simulink model "PVRobusMPC_final"  (R2018a)
settings: Solver=ode2  StartTime=0.0  StopTime=43200  FixedStep=1  RelTol=1e-3  EnableMultiTasking=on
InitFcn:
  | load PV_model_data
StopFcn:
  | save results Lambda_UV01 T_PV_Reference Tm_f01 Pout01 Tamb Time
  | clear all
  | load results
  | figure
  | subplot(3,1,1)
  | plot(Time./3600,T_PV_Reference,Time./3600,Tm_f01)
  | legend('PV Temperature Reference','PV Temperature')
  | title('MPC Tracking')
  | ylim([350 380])
  | subplot(3,1,2)
  | plot(Time./3600,Lambda_UV01)
  | ylim([250 450])
  | legend('\lambda_U_V')
  | subplot(3,1,3)
  | plot(Time./3600,Pout01)
  | legend('PV Power')
  | xlabel('Time [hours]')
  | ylabel('Watt')
values from neighbouring files (symbols this model uses):
  Global_tilt_Irr_2_2_12_13_5 = [0.000279 0.000786 0.00115 0.00401 0.0047 0.0102 0.011 0.0195 0.0266 0.0299 0.0338 0.0682 ... (2802 elements, 1401x2)]    [PV_model_data.mat]
  Total_light_absorption_in_polystyren = [0.0148235487596 0.0159326919994 0.0170383922491 0.0181406655151 0.0192395277052 0.0203349946285 0.0214270819969 0.0225158054254 0.0236011804327 0.0246832224425 0.0257619467839 0.0264640052027 ... (1151 elements, 1151x1)]    [PV_model_data.mat]
  Total_light_absorption_in_PV_cell_acrylic = [0.0222539070262 0.0239185757929 0.0255780524095 0.0272323791236 0.0288816001883 0.030525761736 0.0321649116541 0.0337990994657 0.0354283762117 0.0370527943369 0.0386724075795 0.0397267002838 ... (1151 elements, 1151x1)]    [PV_model_data.mat]
libraries: mpclib x256
(part 2 of 72)

== system PVRobusMPC_final/4 x 4 x 4 PV Panel 2/4 x 4 PV Panel 6/4 PV Panel 3 ==
  lambda_IR : Inport
  Tambient : Inport  Port=2
  Wind Speed : Inport  Port=3
  Add1 : Sum  Inputs=++++
  Add3 : Sum  Inputs=++++
  PV Panel 5 : Subsystem
  PV Panel 6 : Subsystem
  PV Panel 7 : Subsystem
  PV Panel 8 : Subsystem
  Vout : Outport
  Pout : Outport  Port=2
  wires:
  PV Panel 5/2(Pout) -> Add3/1
  PV Panel 8/2(Pout) -> Add3/4
  Add1/1 -> Vout/1
  PV Panel 8/1(Vout) -> Add1/4
  PV Panel 6/1(Vout) -> Add1/2
  lambda_IR/1 -> PV Panel 5/1(Lambda_IR), PV Panel 7/1(Lambda_IR), PV Panel 8/1(Lambda_IR), PV Panel 6/1(Lambda_IR)
  PV Panel 7/2(Pout) -> Add3/3
  Add3/1 -> Pout/1
  Tambient/1 -> PV Panel 7/2(Tambient), PV Panel 8/2(Tambient), PV Panel 6/2(Tambient), PV Panel 5/2(Tambient)
  Wind Speed/1 -> PV Panel 7/3(Wind Speed), PV Panel 8/3(Wind Speed), PV Panel 6/3(Wind Speed), PV Panel 5/3(Wind Speed)
  PV Panel 7/1(Vout) -> Add1/3
  PV Panel 6/2(Pout) -> Add3/2
  PV Panel 5/1(Vout) -> Add1/1

== system PVRobusMPC_final/4 x 4 x 4 PV Panel 2/4 x 4 PV Panel 6/4 PV Panel 4 ==
  lambda_IR : Inport
  Tambient : Inport  Port=2
  Wind Speed : Inport  Port=3
  Add1 : Sum  Inputs=++++
  Add3 : Sum  Inputs=++++
  PV Panel 5 : Subsystem
  PV Panel 6 : Subsystem
  PV Panel 7 : Subsystem
  PV Panel 8 : Subsystem
  Vout : Outport
  Pout : Outport  Port=2
  wires:
  PV Panel 5/1(Vout) -> Add1/1
  PV Panel 6/2(Pout) -> Add3/2
  PV Panel 7/1(Vout) -> Add1/3
  Wind Speed/1 -> PV Panel 5/3(Wind Speed), PV Panel 6/3(Wind Speed), PV Panel 8/3(Wind Speed), PV Panel 7/3(Wind Speed)
  Tambient/1 -> PV Panel 5/2(Tambient), PV Panel 6/2(Tambient), PV Panel 8/2(Tambient), PV Panel 7/2(Tambient)
  Add3/1 -> Pout/1
  PV Panel 7/2(Pout) -> Add3/3
  lambda_IR/1 -> PV Panel 6/1(Lambda_IR), PV Panel 8/1(Lambda_IR), PV Panel 7/1(Lambda_IR), PV Panel 5/1(Lambda_IR)
  PV Panel 6/1(Vout) -> Add1/2
  PV Panel 8/1(Vout) -> Add1/4
  Add1/1 -> Vout/1
  PV Panel 8/2(Pout) -> Add3/4
  PV Panel 5/2(Pout) -> Add3/1

== system PVRobusMPC_final/4 x 4 x 4 PV Panel 2/4 x 4 PV Panel 7/4 PV Panel 1 ==
  lambda_IR : Inport
  Tambient1 : Inport  Port=2
  Wind Speed : Inport  Port=3
  Add : Sum  Inputs=++++
  Add2 : Sum  Inputs=++++
  PV Panel 1 : Subsystem
  PV Panel 2 : Subsystem
  PV Panel 3 : Subsystem
  PV Panel 4 : Subsystem
  Vout : Outport
  Pout : Outport  Port=2
  wires:
  PV Panel 3/2(Pout) -> Add2/3
  lambda_IR/1 -> PV Panel 1/1(Lambda_IR), PV Panel 2/1(Lambda_IR), PV Panel 4/1(Lambda_IR), PV Panel 3/1(Lambda_IR)
  Add/1 -> Vout/1
  PV Panel 1/2(Pout) -> Add2/1
  Tambient1/1 -> PV Panel 1/2(Tambient), PV Panel 2/2(Tambient), PV Panel 3/2(Tambient), PV Panel 4/2(Tambient)
  PV Panel 1/1(Vout) -> Add/1
  PV Panel 4/1(Vout) -> Add/4
  Wind Speed/1 -> PV Panel 1/3(Wind Speed), PV Panel 2/3(Wind Speed), PV Panel 4/3(Wind Speed), PV Panel 3/3(Wind Speed)
  PV Panel 3/1(Vout) -> Add/3
  PV Panel 2/2(Pout) -> Add2/2
  PV Panel 4/2(Pout) -> Add2/4
  PV Panel 2/1(Vout) -> Add/2
  Add2/1 -> Pout/1

== system PVRobusMPC_final/4 x 4 x 4 PV Panel 2/4 x 4 PV Panel 7/4 PV Panel 2 ==
  lambda_IR : Inport
  Tambient : Inport  Port=2
  Wind Speed : Inport  Port=3
  Add1 : Sum  Inputs=++++
  Add3 : Sum  Inputs=++++
  PV Panel 5 : Subsystem
  PV Panel 6 : Subsystem
  PV Panel 7 : Subsystem
  PV Panel 8 : Subsystem
  Vout : Outport
  Pout : Outport  Port=2
  wires:
  PV Panel 5/1(Vout) -> Add1/1
  PV Panel 6/2(Pout) -> Add3/2
  PV Panel 7/1(Vout) -> Add1/3
  Wind Speed/1 -> PV Panel 5/3(Wind Speed), PV Panel 6/3(Wind Speed), PV Panel 8/3(Wind Speed), PV Panel 7/3(Wind Speed)
  Tambient/1 -> PV Panel 5/2(Tambient), PV Panel 6/2(Tambient), PV Panel 8/2(Tambient), PV Panel 7/2(Tambient)
  Add3/1 -> Pout/1
  PV Panel 7/2(Pout) -> Add3/3
  lambda_IR/1 -> PV Panel 6/1(Lambda_IR), PV Panel 8/1(Lambda_IR), PV Panel 7/1(Lambda_IR), PV Panel 5/1(Lambda_IR)
  PV Panel 6/1(Vout) -> Add1/2
  PV Panel 8/1(Vout) -> Add1/4
  Add1/1 -> Vout/1
  PV Panel 8/2(Pout) -> Add3/4
  PV Panel 5/2(Pout) -> Add3/1

== system PVRobusMPC_final/4 x 4 x 4 PV Panel 2/4 x 4 PV Panel 7/4 PV Panel 3 ==
  lambda_IR : Inport
  Tambient : Inport  Port=2
  Wind Speed : Inport  Port=3
  Add1 : Sum  Inputs=++++
  Add3 : Sum  Inputs=++++
  PV Panel 5 : Subsystem
  PV Panel 6 : Subsystem
  PV Panel 7 : Subsystem
  PV Panel 8 : Subsystem
  Vout : Outport
  Pout : Outport  Port=2
  wires:
  PV Panel 5/2(Pout) -> Add3/1
  PV Panel 8/2(Pout) -> Add3/4
  Add1/1 -> Vout/1
  PV Panel 8/1(Vout) -> Add1/4
  PV Panel 6/1(Vout) -> Add1/2
  lambda_IR/1 -> PV Panel 5/1(Lambda_IR), PV Panel 7/1(Lambda_IR), PV Panel 8/1(Lambda_IR), PV Panel 6/1(Lambda_IR)
  PV Panel 7/2(Pout) -> Add3/3
  Add3/1 -> Pout/1
  Tambient/1 -> PV Panel 7/2(Tambient), PV Panel 8/2(Tambient), PV Panel 6/2(Tambient), PV Panel 5/2(Tambient)
  Wind Speed/1 -> PV Panel 7/3(Wind Speed), PV Panel 8/3(Wind Speed), PV Panel 6/3(Wind Speed), PV Panel 5/3(Wind Speed)
  PV Panel 7/1(Vout) -> Add1/3
  PV Panel 6/2(Pout) -> Add3/2
  PV Panel 5/1(Vout) -> Add1/1

== system PVRobusMPC_final/4 x 4 x 4 PV Panel 2/4 x 4 PV Panel 7/4 PV Panel 4 ==
  lambda_IR : Inport
  Tambient : Inport  Port=2
  Wind Speed : Inport  Port=3
  Add1 : Sum  Inputs=++++
  Add3 : Sum  Inputs=++++
  PV Panel 5 : Subsystem
  PV Panel 6 : Subsystem
  PV Panel 7 : Subsystem
  PV Panel 8 : Subsystem
  Vout : Outport
  Pout : Outport  Port=2
  wires:
  PV Panel 5/1(Vout) -> Add1/1
  PV Panel 6/2(Pout) -> Add3/2
  PV Panel 7/1(Vout) -> Add1/3
  Wind Speed/1 -> PV Panel 5/3(Wind Speed), PV Panel 6/3(Wind Speed), PV Panel 8/3(Wind Speed), PV Panel 7/3(Wind Speed)
  Tambient/1 -> PV Panel 5/2(Tambient), PV Panel 6/2(Tambient), PV Panel 8/2(Tambient), PV Panel 7/2(Tambient)
  Add3/1 -> Pout/1
  PV Panel 7/2(Pout) -> Add3/3
  lambda_IR/1 -> PV Panel 6/1(Lambda_IR), PV Panel 8/1(Lambda_IR), PV Panel 7/1(Lambda_IR), PV Panel 5/1(Lambda_IR)
  PV Panel 6/1(Vout) -> Add1/2
  PV Panel 8/1(Vout) -> Add1/4
  Add1/1 -> Vout/1
  PV Panel 8/2(Pout) -> Add3/4
  PV Panel 5/2(Pout) -> Add3/1

== system PVRobusMPC_final/4 x 4 x 4 PV Panel 2/4 x 4 PV Panel 8/4 PV Panel 1 ==
  lambda_IR : Inport
  Tambient1 : Inport  Port=2
  Wind Speed : Inport  Port=3
  Add : Sum  Inputs=++++
  Add2 : Sum  Inputs=++++
  PV Panel 1 : Subsystem
  PV Panel 2 : Subsystem
  PV Panel 3 : Subsystem
  PV Panel 4 : Subsystem
  Vout : Outport
  Pout : Outport  Port=2
  wires:
  Add2/1 -> Pout/1
  PV Panel 2/1(Vout) -> Add/2
  PV Panel 4/2(Pout) -> Add2/4
  PV Panel 2/2(Pout) -> Add2/2
  PV Panel 3/1(Vout) -> Add/3
  Wind Speed/1 -> PV Panel 3/3(Wind Speed), PV Panel 4/3(Wind Speed), PV Panel 2/3(Wind Speed), PV Panel 1/3(Wind Speed)
  PV Panel 4/1(Vout) -> Add/4
  PV Panel 1/1(Vout) -> Add/1
  Tambient1/1 -> PV Panel 4/2(Tambient), PV Panel 3/2(Tambient), PV Panel 2/2(Tambient), PV Panel 1/2(Tambient)
  PV Panel 1/2(Pout) -> Add2/1
  Add/1 -> Vout/1
  lambda_IR/1 -> PV Panel 3/1(Lambda_IR), PV Panel 4/1(Lambda_IR), PV Panel 2/1(Lambda_IR), PV Panel 1/1(Lambda_IR)
  PV Panel 3/2(Pout) -> Add2/3

== system PVRobusMPC_final/4 x 4 x 4 PV Panel 2/4 x 4 PV Panel 8/4 PV Panel 2 ==
  lambda_IR : Inport
  Tambient : Inport  Port=2
  Wind Speed : Inport  Port=3
  Add1 : Sum  Inputs=++++
  Add3 : Sum  Inputs=++++
  PV Panel 5 : Subsystem
  PV Panel 6 : Subsystem
  PV Panel 7 : Subsystem
  PV Panel 8 : Subsystem
  Vout : Outport
  Pout : Outport  Port=2
  wires:
  PV Panel 5/2(Pout) -> Add3/1
  PV Panel 8/2(Pout) -> Add3/4
  Add1/1 -> Vout/1
  PV Panel 8/1(Vout) -> Add1/4
  PV Panel 6/1(Vout) -> Add1/2
  lambda_IR/1 -> PV Panel 5/1(Lambda_IR), PV Panel 7/1(Lambda_IR), PV Panel 8/1(Lambda_IR), PV Panel 6/1(Lambda_IR)
  PV Panel 7/2(Pout) -> Add3/3
  Add3/1 -> Pout/1
  Tambient/1 -> PV Panel 7/2(Tambient), PV Panel 8/2(Tambient), PV Panel 6/2(Tambient), PV Panel 5/2(Tambient)
  Wind Speed/1 -> PV Panel 7/3(Wind Speed), PV Panel 8/3(Wind Speed), PV Panel 6/3(Wind Speed), PV Panel 5/3(Wind Speed)
  PV Panel 7/1(Vout) -> Add1/3
  PV Panel 6/2(Pout) -> Add3/2
  PV Panel 5/1(Vout) -> Add1/1

== system PVRobusMPC_final/4 x 4 x 4 PV Panel 2/4 x 4 PV Panel 8/4 PV Panel 3 ==
  lambda_IR : Inport
  Tambient : Inport  Port=2
  Wind Speed : Inport  Port=3
  Add1 : Sum  Inputs=++++
  Add3 : Sum  Inputs=++++
  PV Panel 5 : Subsystem
  PV Panel 6 : Subsystem
  PV Panel 7 : Subsystem
  PV Panel 8 : Subsystem
  Vout : Outport
  Pout : Outport  Port=2
  wires:
  PV Panel 5/1(Vout) -> Add1/1
  PV Panel 6/2(Pout) -> Add3/2
  PV Panel 7/1(Vout) -> Add1/3
  Wind Speed/1 -> PV Panel 5/3(Wind Speed), PV Panel 6/3(Wind Speed), PV Panel 8/3(Wind Speed), PV Panel 7/3(Wind Speed)
  Tambient/1 -> PV Panel 5/2(Tambient), PV Panel 6/2(Tambient), PV Panel 8/2(Tambient), PV Panel 7/2(Tambient)
  Add3/1 -> Pout/1
  PV Panel 7/2(Pout) -> Add3/3
  lambda_IR/1 -> PV Panel 6/1(Lambda_IR), PV Panel 8/1(Lambda_IR), PV Panel 7/1(Lambda_IR), PV Panel 5/1(Lambda_IR)
  PV Panel 6/1(Vout) -> Add1/2
  PV Panel 8/1(Vout) -> Add1/4
  Add1/1 -> Vout/1
  PV Panel 8/2(Pout) -> Add3/4
  PV Panel 5/2(Pout) -> Add3/1

== system PVRobusMPC_final/4 x 4 x 4 PV Panel 2/4 x 4 PV Panel 8/4 PV Panel 4 ==
  lambda_IR : Inport
  Tambient : Inport  Port=2
  Wind Speed : Inport  Port=3
  Add1 : Sum  Inputs=++++
  Add3 : Sum  Inputs=++++
  PV Panel 5 : Subsystem
  PV Panel 6 : Subsystem
  PV Panel 7 : Subsystem
  PV Panel 8 : Subsystem
  Vout : Outport
  Pout : Outport  Port=2
  wires:
  PV Panel 5/2(Pout) -> Add3/1
  PV Panel 8/2(Pout) -> Add3/4
  Add1/1 -> Vout/1
  PV Panel 8/1(Vout) -> Add1/4
  PV Panel 6/1(Vout) -> Add1/2
  lambda_IR/1 -> PV Panel 5/1(Lambda_IR), PV Panel 7/1(Lambda_IR), PV Panel 8/1(Lambda_IR), PV Panel 6/1(Lambda_IR)
  PV Panel 7/2(Pout) -> Add3/3
  Add3/1 -> Pout/1
  Tambient/1 -> PV Panel 7/2(Tambient), PV Panel 8/2(Tambient), PV Panel 6/2(Tambient), PV Panel 5/2(Tambient)
  Wind Speed/1 -> PV Panel 7/3(Wind Speed), PV Panel 8/3(Wind Speed), PV Panel 6/3(Wind Speed), PV Panel 5/3(Wind Speed)
  PV Panel 7/1(Vout) -> Add1/3
  PV Panel 6/2(Pout) -> Add3/2
  PV Panel 5/1(Vout) -> Add1/1

== system PVRobusMPC_final/4 x 4 x 4 PV Panel 3/4 x 4 PV Panel 5/4 PV Panel 1 ==
  lambda_IR : Inport
  Tambient1 : Inport  Port=2
  Wind Speed : Inport  Port=3
  Add : Sum  Inputs=++++
  Add2 : Sum  Inputs=++++
  PV Panel 1 : Subsystem
  PV Panel 2 : Subsystem
  PV Panel 3 : Subsystem
  PV Panel 4 : Subsystem
  Vout : Outport
  Pout : Outport  Port=2
  wires:
  Add2/1 -> Pout/1
  PV Panel 2/1(Vout) -> Add/2
  PV Panel 4/2(Pout) -> Add2/4
  PV Panel 2/2(Pout) -> Add2/2
  PV Panel 3/1(Vout) -> Add/3
  Wind Speed/1 -> PV Panel 3/3(Wind Speed), PV Panel 4/3(Wind Speed), PV Panel 2/3(Wind Speed), PV Panel 1/3(Wind Speed)
  PV Panel 4/1(Vout) -> Add/4
  PV Panel 1/1(Vout) -> Add/1
  Tambient1/1 -> PV Panel 4/2(Tambient), PV Panel 3/2(Tambient), PV Panel 2/2(Tambient), PV Panel 1/2(Tambient)
  PV Panel 1/2(Pout) -> Add2/1
  Add/1 -> Vout/1
  lambda_IR/1 -> PV Panel 3/1(Lambda_IR), PV Panel 4/1(Lambda_IR), PV Panel 2/1(Lambda_IR), PV Panel 1/1(Lambda_IR)
  PV Panel 3/2(Pout) -> Add2/3

== system PVRobusMPC_final/4 x 4 x 4 PV Panel 3/4 x 4 PV Panel 5/4 PV Panel 2 ==
  lambda_IR : Inport
  Tambient : Inport  Port=2
  Wind Speed : Inport  Port=3
  Add1 : Sum  Inputs=++++
  Add3 : Sum  Inputs=++++
  PV Panel 5 : Subsystem
  PV Panel 6 : Subsystem
  PV Panel 7 : Subsystem
  PV Panel 8 : Subsystem
  Vout : Outport
  Pout : Outport  Port=2
  wires:
  PV Panel 5/2(Pout) -> Add3/1
  PV Panel 8/2(Pout) -> Add3/4
  Add1/1 -> Vout/1
  PV Panel 8/1(Vout) -> Add1/4
  PV Panel 6/1(Vout) -> Add1/2
  lambda_IR/1 -> PV Panel 5/1(Lambda_IR), PV Panel 7/1(Lambda_IR), PV Panel 8/1(Lambda_IR), PV Panel 6/1(Lambda_IR)
  PV Panel 7/2(Pout) -> Add3/3
  Add3/1 -> Pout/1
  Tambient/1 -> PV Panel 7/2(Tambient), PV Panel 8/2(Tambient), PV Panel 6/2(Tambient), PV Panel 5/2(Tambient)
  Wind Speed/1 -> PV Panel 7/3(Wind Speed), PV Panel 8/3(Wind Speed), PV Panel 6/3(Wind Speed), PV Panel 5/3(Wind Speed)
  PV Panel 7/1(Vout) -> Add1/3
  PV Panel 6/2(Pout) -> Add3/2
  PV Panel 5/1(Vout) -> Add1/1

== system PVRobusMPC_final/4 x 4 x 4 PV Panel 3/4 x 4 PV Panel 5/4 PV Panel 3 ==
  lambda_IR : Inport
  Tambient : Inport  Port=2
  Wind Speed : Inport  Port=3
  Add1 : Sum  Inputs=++++
  Add3 : Sum  Inputs=++++
  PV Panel 5 : Subsystem
  PV Panel 6 : Subsystem
  PV Panel 7 : Subsystem
  PV Panel 8 : Subsystem
  Vout : Outport
  Pout : Outport  Port=2
  wires:
  PV Panel 5/1(Vout) -> Add1/1
  PV Panel 6/2(Pout) -> Add3/2
  PV Panel 7/1(Vout) -> Add1/3
  Wind Speed/1 -> PV Panel 5/3(Wind Speed), PV Panel 6/3(Wind Speed), PV Panel 8/3(Wind Speed), PV Panel 7/3(Wind Speed)
  Tambient/1 -> PV Panel 5/2(Tambient), PV Panel 6/2(Tambient), PV Panel 8/2(Tambient), PV Panel 7/2(Tambient)
  Add3/1 -> Pout/1
  PV Panel 7/2(Pout) -> Add3/3
  lambda_IR/1 -> PV Panel 6/1(Lambda_IR), PV Panel 8/1(Lambda_IR), PV Panel 7/1(Lambda_IR), PV Panel 5/1(Lambda_IR)
  PV Panel 6/1(Vout) -> Add1/2
  PV Panel 8/1(Vout) -> Add1/4
  Add1/1 -> Vout/1
  PV Panel 8/2(Pout) -> Add3/4
  PV Panel 5/2(Pout) -> Add3/1

== system PVRobusMPC_final/4 x 4 x 4 PV Panel 3/4 x 4 PV Panel 5/4 PV Panel 4 ==
  lambda_IR : Inport
  Tambient : Inport  Port=2
  Wind Speed : Inport  Port=3
  Add1 : Sum  Inputs=++++
  Add3 : Sum  Inputs=++++
  PV Panel 5 : Subsystem
  PV Panel 6 : Subsystem
  PV Panel 7 : Subsystem
  PV Panel 8 : Subsystem
  Vout : Outport
  Pout : Outport  Port=2
  wires:
  PV Panel 5/2(Pout) -> Add3/1
  PV Panel 8/2(Pout) -> Add3/4
  Add1/1 -> Vout/1
  PV Panel 8/1(Vout) -> Add1/4
  PV Panel 6/1(Vout) -> Add1/2
  lambda_IR/1 -> PV Panel 5/1(Lambda_IR), PV Panel 7/1(Lambda_IR), PV Panel 8/1(Lambda_IR), PV Panel 6/1(Lambda_IR)
  PV Panel 7/2(Pout) -> Add3/3
  Add3/1 -> Pout/1
  Tambient/1 -> PV Panel 7/2(Tambient), PV Panel 8/2(Tambient), PV Panel 6/2(Tambient), PV Panel 5/2(Tambient)
  Wind Speed/1 -> PV Panel 7/3(Wind Speed), PV Panel 8/3(Wind Speed), PV Panel 6/3(Wind Speed), PV Panel 5/3(Wind Speed)
  PV Panel 7/1(Vout) -> Add1/3
  PV Panel 6/2(Pout) -> Add3/2
  PV Panel 5/1(Vout) -> Add1/1

== system PVRobusMPC_final/4 x 4 x 4 PV Panel 3/4 x 4 PV Panel 6/4 PV Panel 1 ==
  lambda_IR : Inport
  Tambient1 : Inport  Port=2
  Wind Speed : Inport  Port=3
  Add : Sum  Inputs=++++
  Add2 : Sum  Inputs=++++
  PV Panel 1 : Subsystem
  PV Panel 2 : Subsystem
  PV Panel 3 : Subsystem
  PV Panel 4 : Subsystem
  Vout : Outport
  Pout : Outport  Port=2
  wires:
  Add2/1 -> Pout/1
  PV Panel 2/1(Vout) -> Add/2
  PV Panel 4/2(Pout) -> Add2/4
  PV Panel 2/2(Pout) -> Add2/2
  PV Panel 3/1(Vout) -> Add/3
  Wind Speed/1 -> PV Panel 3/3(Wind Speed), PV Panel 4/3(Wind Speed), PV Panel 2/3(Wind Speed), PV Panel 1/3(Wind Speed)
  PV Panel 4/1(Vout) -> Add/4
  PV Panel 1/1(Vout) -> Add/1
  Tambient1/1 -> PV Panel 4/2(Tambient), PV Panel 3/2(Tambient), PV Panel 2/2(Tambient), PV Panel 1/2(Tambient)
  PV Panel 1/2(Pout) -> Add2/1
  Add/1 -> Vout/1
  lambda_IR/1 -> PV Panel 3/1(Lambda_IR), PV Panel 4/1(Lambda_IR), PV Panel 2/1(Lambda_IR), PV Panel 1/1(Lambda_IR)
  PV Panel 3/2(Pout) -> Add2/3

== system PVRobusMPC_final/4 x 4 x 4 PV Panel 3/4 x 4 PV Panel 6/4 PV Panel 2 ==
  lambda_IR : Inport
  Tambient : Inport  Port=2
  Wind Speed : Inport  Port=3
  Add1 : Sum  Inputs=++++
  Add3 : Sum  Inputs=++++
  PV Panel 5 : Subsystem
  PV Panel 6 : Subsystem
  PV Panel 7 : Subsystem
  PV Panel 8 : Subsystem
  Vout : Outport
  Pout : Outport  Port=2
  wires:
  PV Panel 5/2(Pout) -> Add3/1
  PV Panel 8/2(Pout) -> Add3/4
  Add1/1 -> Vout/1
  PV Panel 8/1(Vout) -> Add1/4
  PV Panel 6/1(Vout) -> Add1/2
  lambda_IR/1 -> PV Panel 5/1(Lambda_IR), PV Panel 7/1(Lambda_IR), PV Panel 8/1(Lambda_IR), PV Panel 6/1(Lambda_IR)
  PV Panel 7/2(Pout) -> Add3/3
  Add3/1 -> Pout/1
  Tambient/1 -> PV Panel 7/2(Tambient), PV Panel 8/2(Tambient), PV Panel 6/2(Tambient), PV Panel 5/2(Tambient)
  Wind Speed/1 -> PV Panel 7/3(Wind Speed), PV Panel 8/3(Wind Speed), PV Panel 6/3(Wind Speed), PV Panel 5/3(Wind Speed)
  PV Panel 7/1(Vout) -> Add1/3
  PV Panel 6/2(Pout) -> Add3/2
  PV Panel 5/1(Vout) -> Add1/1

== system PVRobusMPC_final/4 x 4 x 4 PV Panel 3/4 x 4 PV Panel 6/4 PV Panel 3 ==
  lambda_IR : Inport
  Tambient : Inport  Port=2
  Wind Speed : Inport  Port=3
  Add1 : Sum  Inputs=++++
  Add3 : Sum  Inputs=++++
  PV Panel 5 : Subsystem
  PV Panel 6 : Subsystem
  PV Panel 7 : Subsystem
  PV Panel 8 : Subsystem
  Vout : Outport
  Pout : Outport  Port=2
  wires:
  PV Panel 5/1(Vout) -> Add1/1
  PV Panel 6/2(Pout) -> Add3/2
  PV Panel 7/1(Vout) -> Add1/3
  Wind Speed/1 -> PV Panel 5/3(Wind Speed), PV Panel 6/3(Wind Speed), PV Panel 8/3(Wind Speed), PV Panel 7/3(Wind Speed)
  Tambient/1 -> PV Panel 5/2(Tambient), PV Panel 6/2(Tambient), PV Panel 8/2(Tambient), PV Panel 7/2(Tambient)
  Add3/1 -> Pout/1
  PV Panel 7/2(Pout) -> Add3/3
  lambda_IR/1 -> PV Panel 6/1(Lambda_IR), PV Panel 8/1(Lambda_IR), PV Panel 7/1(Lambda_IR), PV Panel 5/1(Lambda_IR)
  PV Panel 6/1(Vout) -> Add1/2
  PV Panel 8/1(Vout) -> Add1/4
  Add1/1 -> Vout/1
  PV Panel 8/2(Pout) -> Add3/4
  PV Panel 5/2(Pout) -> Add3/1

== system PVRobusMPC_final/4 x 4 x 4 PV Panel 3/4 x 4 PV Panel 6/4 PV Panel 4 ==
  lambda_IR : Inport
  Tambient : Inport  Port=2
  Wind Speed : Inport  Port=3
  Add1 : Sum  Inputs=++++
  Add3 : Sum  Inputs=++++
  PV Panel 5 : Subsystem
  PV Panel 6 : Subsystem
  PV Panel 7 : Subsystem
  PV Panel 8 : Subsystem
  Vout : Outport
  Pout : Outport  Port=2
  wires:
  PV Panel 5/2(Pout) -> Add3/1
  PV Panel 8/2(Pout) -> Add3/4
  Add1/1 -> Vout/1
  PV Panel 8/1(Vout) -> Add1/4
  PV Panel 6/1(Vout) -> Add1/2
  lambda_IR/1 -> PV Panel 5/1(Lambda_IR), PV Panel 7/1(Lambda_IR), PV Panel 8/1(Lambda_IR), PV Panel 6/1(Lambda_IR)
  PV Panel 7/2(Pout) -> Add3/3
  Add3/1 -> Pout/1
  Tambient/1 -> PV Panel 7/2(Tambient), PV Panel 8/2(Tambient), PV Panel 6/2(Tambient), PV Panel 5/2(Tambient)
  Wind Speed/1 -> PV Panel 7/3(Wind Speed), PV Panel 8/3(Wind Speed), PV Panel 6/3(Wind Speed), PV Panel 5/3(Wind Speed)
  PV Panel 7/1(Vout) -> Add1/3
  PV Panel 6/2(Pout) -> Add3/2
  PV Panel 5/1(Vout) -> Add1/1

== system PVRobusMPC_final/4 x 4 x 4 PV Panel 3/4 x 4 PV Panel 7/4 PV Panel 1 ==
  lambda_IR : Inport
  Tambient1 : Inport  Port=2
  Wind Speed : Inport  Port=3
  Add : Sum  Inputs=++++
  Add2 : Sum  Inputs=++++
  PV Panel 1 : Subsystem
  PV Panel 2 : Subsystem
  PV Panel 3 : Subsystem
  PV Panel 4 : Subsystem
  Vout : Outport
  Pout : Outport  Port=2
  wires:
  Add2/1 -> Pout/1
  PV Panel 2/1(Vout) -> Add/2
  PV Panel 4/2(Pout) -> Add2/4
  PV Panel 2/2(Pout) -> Add2/2
  PV Panel 3/1(Vout) -> Add/3
  Wind Speed/1 -> PV Panel 3/3(Wind Speed), PV Panel 4/3(Wind Speed), PV Panel 2/3(Wind Speed), PV Panel 1/3(Wind Speed)
  PV Panel 4/1(Vout) -> Add/4
  PV Panel 1/1(Vout) -> Add/1
  Tambient1/1 -> PV Panel 4/2(Tambient), PV Panel 3/2(Tambient), PV Panel 2/2(Tambient), PV Panel 1/2(Tambient)
  PV Panel 1/2(Pout) -> Add2/1
  Add/1 -> Vout/1
  lambda_IR/1 -> PV Panel 3/1(Lambda_IR), PV Panel 4/1(Lambda_IR), PV Panel 2/1(Lambda_IR), PV Panel 1/1(Lambda_IR)
  PV Panel 3/2(Pout) -> Add2/3

== system PVRobusMPC_final/4 x 4 x 4 PV Panel 3/4 x 4 PV Panel 7/4 PV Panel 2 ==
  lambda_IR : Inport
  Tambient : Inport  Port=2
  Wind Speed : Inport  Port=3
  Add1 : Sum  Inputs=++++
  Add3 : Sum  Inputs=++++
  PV Panel 5 : Subsystem
  PV Panel 6 : Subsystem
  PV Panel 7 : Subsystem
  PV Panel 8 : Subsystem
  Vout : Outport
  Pout : Outport  Port=2
  wires:
  PV Panel 5/2(Pout) -> Add3/1
  PV Panel 8/2(Pout) -> Add3/4
  Add1/1 -> Vout/1
  PV Panel 8/1(Vout) -> Add1/4
  PV Panel 6/1(Vout) -> Add1/2
  lambda_IR/1 -> PV Panel 5/1(Lambda_IR), PV Panel 7/1(Lambda_IR), PV Panel 8/1(Lambda_IR), PV Panel 6/1(Lambda_IR)
  PV Panel 7/2(Pout) -> Add3/3
  Add3/1 -> Pout/1
  Tambient/1 -> PV Panel 7/2(Tambient), PV Panel 8/2(Tambient), PV Panel 6/2(Tambient), PV Panel 5/2(Tambient)
  Wind Speed/1 -> PV Panel 7/3(Wind Speed), PV Panel 8/3(Wind Speed), PV Panel 6/3(Wind Speed), PV Panel 5/3(Wind Speed)
  PV Panel 7/1(Vout) -> Add1/3
  PV Panel 6/2(Pout) -> Add3/2
  PV Panel 5/1(Vout) -> Add1/1

== system PVRobusMPC_final/4 x 4 x 4 PV Panel 3/4 x 4 PV Panel 7/4 PV Panel 3 ==
  lambda_IR : Inport
  Tambient : Inport  Port=2
  Wind Speed : Inport  Port=3
  Add1 : Sum  Inputs=++++
  Add3 : Sum  Inputs=++++
  PV Panel 5 : Subsystem
  PV Panel 6 : Subsystem
  PV Panel 7 : Subsystem
  PV Panel 8 : Subsystem
  Vout : Outport
  Pout : Outport  Port=2
  wires:
  PV Panel 5/1(Vout) -> Add1/1
  PV Panel 6/2(Pout) -> Add3/2
  PV Panel 7/1(Vout) -> Add1/3
  Wind Speed/1 -> PV Panel 5/3(Wind Speed), PV Panel 6/3(Wind Speed), PV Panel 8/3(Wind Speed), PV Panel 7/3(Wind Speed)
  Tambient/1 -> PV Panel 5/2(Tambient), PV Panel 6/2(Tambient), PV Panel 8/2(Tambient), PV Panel 7/2(Tambient)
  Add3/1 -> Pout/1
  PV Panel 7/2(Pout) -> Add3/3
  lambda_IR/1 -> PV Panel 6/1(Lambda_IR), PV Panel 8/1(Lambda_IR), PV Panel 7/1(Lambda_IR), PV Panel 5/1(Lambda_IR)
  PV Panel 6/1(Vout) -> Add1/2
  PV Panel 8/1(Vout) -> Add1/4
  Add1/1 -> Vout/1
  PV Panel 8/2(Pout) -> Add3/4
  PV Panel 5/2(Pout) -> Add3/1

== system PVRobusMPC_final/4 x 4 x 4 PV Panel 3/4 x 4 PV Panel 7/4 PV Panel 4 ==
  lambda_IR : Inport
  Tambient : Inport  Port=2
  Wind Speed : Inport  Port=3
  Add1 : Sum  Inputs=++++
  Add3 : Sum  Inputs=++++
  PV Panel 5 : Subsystem
  PV Panel 6 : Subsystem
  PV Panel 7 : Subsystem
  PV Panel 8 : Subsystem
  Vout : Outport
  Pout : Outport  Port=2
  wires:
  PV Panel 5/2(Pout) -> Add3/1
  PV Panel 8/2(Pout) -> Add3/4
  Add1/1 -> Vout/1
  PV Panel 8/1(Vout) -> Add1/4
  PV Panel 6/1(Vout) -> Add1/2
  lambda_IR/1 -> PV Panel 5/1(Lambda_IR), PV Panel 7/1(Lambda_IR), PV Panel 8/1(Lambda_IR), PV Panel 6/1(Lambda_IR)
  PV Panel 7/2(Pout) -> Add3/3
  Add3/1 -> Pout/1
  Tambient/1 -> PV Panel 7/2(Tambient), PV Panel 8/2(Tambient), PV Panel 6/2(Tambient), PV Panel 5/2(Tambient)
  Wind Speed/1 -> PV Panel 7/3(Wind Speed), PV Panel 8/3(Wind Speed), PV Panel 6/3(Wind Speed), PV Panel 5/3(Wind Speed)
  PV Panel 7/1(Vout) -> Add1/3
  PV Panel 6/2(Pout) -> Add3/2
  PV Panel 5/1(Vout) -> Add1/1

== system PVRobusMPC_final/4 x 4 x 4 PV Panel 3/4 x 4 PV Panel 8/4 PV Panel 1 ==
  lambda_IR : Inport
  Tambient1 : Inport  Port=2
  Wind Speed : Inport  Port=3
  Add : Sum  Inputs=++++
  Add2 : Sum  Inputs=++++
  PV Panel 1 : Subsystem
  PV Panel 2 : Subsystem
  PV Panel 3 : Subsystem
  PV Panel 4 : Subsystem
  Vout : Outport
  Pout : Outport  Port=2
  wires:
  PV Panel 3/2(Pout) -> Add2/3
  lambda_IR/1 -> PV Panel 1/1(Lambda_IR), PV Panel 2/1(Lambda_IR), PV Panel 4/1(Lambda_IR), PV Panel 3/1(Lambda_IR)
  Add/1 -> Vout/1
  PV Panel 1/2(Pout) -> Add2/1
  Tambient1/1 -> PV Panel 1/2(Tambient), PV Panel 2/2(Tambient), PV Panel 3/2(Tambient), PV Panel 4/2(Tambient)
  PV Panel 1/1(Vout) -> Add/1
  PV Panel 4/1(Vout) -> Add/4
  Wind Speed/1 -> PV Panel 1/3(Wind Speed), PV Panel 2/3(Wind Speed), PV Panel 4/3(Wind Speed), PV Panel 3/3(Wind Speed)
  PV Panel 3/1(Vout) -> Add/3
  PV Panel 2/2(Pout) -> Add2/2
  PV Panel 4/2(Pout) -> Add2/4
  PV Panel 2/1(Vout) -> Add/2
  Add2/1 -> Pout/1

== system PVRobusMPC_final/4 x 4 x 4 PV Panel 3/4 x 4 PV Panel 8/4 PV Panel 2 ==
  lambda_IR : Inport
  Tambient : Inport  Port=2
  Wind Speed : Inport  Port=3
  Add1 : Sum  Inputs=++++
  Add3 : Sum  Inputs=++++
  PV Panel 5 : Subsystem
  PV Panel 6 : Subsystem
  PV Panel 7 : Subsystem
  PV Panel 8 : Subsystem
  Vout : Outport
  Pout : Outport  Port=2
  wires:
  PV Panel 5/1(Vout) -> Add1/1
  PV Panel 6/2(Pout) -> Add3/2
  PV Panel 7/1(Vout) -> Add1/3
  Wind Speed/1 -> PV Panel 5/3(Wind Speed), PV Panel 6/3(Wind Speed), PV Panel 8/3(Wind Speed), PV Panel 7/3(Wind Speed)
  Tambient/1 -> PV Panel 5/2(Tambient), PV Panel 6/2(Tambient), PV Panel 8/2(Tambient), PV Panel 7/2(Tambient)
  Add3/1 -> Pout/1
  PV Panel 7/2(Pout) -> Add3/3
  lambda_IR/1 -> PV Panel 6/1(Lambda_IR), PV Panel 8/1(Lambda_IR), PV Panel 7/1(Lambda_IR), PV Panel 5/1(Lambda_IR)
  PV Panel 6/1(Vout) -> Add1/2
  PV Panel 8/1(Vout) -> Add1/4
  Add1/1 -> Vout/1
  PV Panel 8/2(Pout) -> Add3/4
  PV Panel 5/2(Pout) -> Add3/1

== system PVRobusMPC_final/4 x 4 x 4 PV Panel 3/4 x 4 PV Panel 8/4 PV Panel 3 ==
  lambda_IR : Inport
  Tambient : Inport  Port=2
  Wind Speed : Inport  Port=3
  Add1 : Sum  Inputs=++++
  Add3 : Sum  Inputs=++++
  PV Panel 5 : Subsystem
  PV Panel 6 : Subsystem
  PV Panel 7 : Subsystem
  PV Panel 8 : Subsystem
  Vout : Outport
  Pout : Outport  Port=2
  wires:
  PV Panel 5/2(Pout) -> Add3/1
  PV Panel 8/2(Pout) -> Add3/4
  Add1/1 -> Vout/1
  PV Panel 8/1(Vout) -> Add1/4
  PV Panel 6/1(Vout) -> Add1/2
  lambda_IR/1 -> PV Panel 5/1(Lambda_IR), PV Panel 7/1(Lambda_IR), PV Panel 8/1(Lambda_IR), PV Panel 6/1(Lambda_IR)
  PV Panel 7/2(Pout) -> Add3/3
  Add3/1 -> Pout/1
  Tambient/1 -> PV Panel 7/2(Tambient), PV Panel 8/2(Tambient), PV Panel 6/2(Tambient), PV Panel 5/2(Tambient)
  Wind Speed/1 -> PV Panel 7/3(Wind Speed), PV Panel 8/3(Wind Speed), PV Panel 6/3(Wind Speed), PV Panel 5/3(Wind Speed)
  PV Panel 7/1(Vout) -> Add1/3
  PV Panel 6/2(Pout) -> Add3/2
  PV Panel 5/1(Vout) -> Add1/1

== system PVRobusMPC_final/4 x 4 x 4 PV Panel 3/4 x 4 PV Panel 8/4 PV Panel 4 ==
  lambda_IR : Inport
  Tambient : Inport  Port=2
  Wind Speed : Inport  Port=3
  Add1 : Sum  Inputs=++++
  Add3 : Sum  Inputs=++++
  PV Panel 5 : Subsystem
  PV Panel 6 : Subsystem
  PV Panel 7 : Subsystem
  PV Panel 8 : Subsystem
  Vout : Outport
  Pout : Outport  Port=2
  wires:
  PV Panel 5/1(Vout) -> Add1/1
  PV Panel 6/2(Pout) -> Add3/2
  PV Panel 7/1(Vout) -> Add1/3
  Wind Speed/1 -> PV Panel 5/3(Wind Speed), PV Panel 6/3(Wind Speed), PV Panel 8/3(Wind Speed), PV Panel 7/3(Wind Speed)
  Tambient/1 -> PV Panel 5/2(Tambient), PV Panel 6/2(Tambient), PV Panel 8/2(Tambient), PV Panel 7/2(Tambient)
  Add3/1 -> Pout/1
  PV Panel 7/2(Pout) -> Add3/3
  lambda_IR/1 -> PV Panel 6/1(Lambda_IR), PV Panel 8/1(Lambda_IR), PV Panel 7/1(Lambda_IR), PV Panel 5/1(Lambda_IR)
  PV Panel 6/1(Vout) -> Add1/2
  PV Panel 8/1(Vout) -> Add1/4
  Add1/1 -> Vout/1
  PV Panel 8/2(Pout) -> Add3/4
  PV Panel 5/2(Pout) -> Add3/1

== system PVRobusMPC_final/4 x 4 x 4 PV Panel 4/4 x 4 PV Panel 5/4 PV Panel 1 ==
  lambda_IR : Inport
  Tambient1 : Inport  Port=2
  Wind Speed : Inport  Port=3
  Add : Sum  Inputs=++++
  Add2 : Sum  Inputs=++++
  PV Panel 1 : Subsystem
  PV Panel 2 : Subsystem
  PV Panel 3 : Subsystem
  PV Panel 4 : Subsystem
  Vout : Outport
  Pout : Outport  Port=2
  wires:
  PV Panel 3/2(Pout) -> Add2/3
  lambda_IR/1 -> PV Panel 1/1(Lambda_IR), PV Panel 2/1(Lambda_IR), PV Panel 4/1(Lambda_IR), PV Panel 3/1(Lambda_IR)
  Add/1 -> Vout/1
  PV Panel 1/2(Pout) -> Add2/1
  Tambient1/1 -> PV Panel 1/2(Tambient), PV Panel 2/2(Tambient), PV Panel 3/2(Tambient), PV Panel 4/2(Tambient)
  PV Panel 1/1(Vout) -> Add/1
  PV Panel 4/1(Vout) -> Add/4
  Wind Speed/1 -> PV Panel 1/3(Wind Speed), PV Panel 2/3(Wind Speed), PV Panel 4/3(Wind Speed), PV Panel 3/3(Wind Speed)
  PV Panel 3/1(Vout) -> Add/3
  PV Panel 2/2(Pout) -> Add2/2
  PV Panel 4/2(Pout) -> Add2/4
  PV Panel 2/1(Vout) -> Add/2
  Add2/1 -> Pout/1

== system PVRobusMPC_final/4 x 4 x 4 PV Panel 4/4 x 4 PV Panel 5/4 PV Panel 2 ==
  lambda_IR : Inport
  Tambient : Inport  Port=2
  Wind Speed : Inport  Port=3
  Add1 : Sum  Inputs=++++
  Add3 : Sum  Inputs=++++
  PV Panel 5 : Subsystem
  PV Panel 6 : Subsystem
  PV Panel 7 : Subsystem
  PV Panel 8 : Subsystem
  Vout : Outport
  Pout : Outport  Port=2
  wires:
  PV Panel 5/1(Vout) -> Add1/1
  PV Panel 6/2(Pout) -> Add3/2
  PV Panel 7/1(Vout) -> Add1/3
  Wind Speed/1 -> PV Panel 5/3(Wind Speed), PV Panel 6/3(Wind Speed), PV Panel 8/3(Wind Speed), PV Panel 7/3(Wind Speed)
  Tambient/1 -> PV Panel 5/2(Tambient), PV Panel 6/2(Tambient), PV Panel 8/2(Tambient), PV Panel 7/2(Tambient)
  Add3/1 -> Pout/1
  PV Panel 7/2(Pout) -> Add3/3
  lambda_IR/1 -> PV Panel 6/1(Lambda_IR), PV Panel 8/1(Lambda_IR), PV Panel 7/1(Lambda_IR), PV Panel 5/1(Lambda_IR)
  PV Panel 6/1(Vout) -> Add1/2
  PV Panel 8/1(Vout) -> Add1/4
  Add1/1 -> Vout/1
  PV Panel 8/2(Pout) -> Add3/4
  PV Panel 5/2(Pout) -> Add3/1

== system PVRobusMPC_final/4 x 4 x 4 PV Panel 4/4 x 4 PV Panel 5/4 PV Panel 3 ==
  lambda_IR : Inport
  Tambient : Inport  Port=2
  Wind Speed : Inport  Port=3
  Add1 : Sum  Inputs=++++
  Add3 : Sum  Inputs=++++
  PV Panel 5 : Subsystem
  PV Panel 6 : Subsystem
  PV Panel 7 : Subsystem
  PV Panel 8 : Subsystem
  Vout : Outport
  Pout : Outport  Port=2
  wires:
  PV Panel 5/2(Pout) -> Add3/1
  PV Panel 8/2(Pout) -> Add3/4
  Add1/1 -> Vout/1
  PV Panel 8/1(Vout) -> Add1/4
  PV Panel 6/1(Vout) -> Add1/2
  lambda_IR/1 -> PV Panel 5/1(Lambda_IR), PV Panel 7/1(Lambda_IR), PV Panel 8/1(Lambda_IR), PV Panel 6/1(Lambda_IR)
  PV Panel 7/2(Pout) -> Add3/3
  Add3/1 -> Pout/1
  Tambient/1 -> PV Panel 7/2(Tambient), PV Panel 8/2(Tambient), PV Panel 6/2(Tambient), PV Panel 5/2(Tambient)
  Wind Speed/1 -> PV Panel 7/3(Wind Speed), PV Panel 8/3(Wind Speed), PV Panel 6/3(Wind Speed), PV Panel 5/3(Wind Speed)
  PV Panel 7/1(Vout) -> Add1/3
  PV Panel 6/2(Pout) -> Add3/2
  PV Panel 5/1(Vout) -> Add1/1

== system PVRobusMPC_final/4 x 4 x 4 PV Panel 4/4 x 4 PV Panel 5/4 PV Panel 4 ==
  lambda_IR : Inport
  Tambient : Inport  Port=2
  Wind Speed : Inport  Port=3
  Add1 : Sum  Inputs=++++
  Add3 : Sum  Inputs=++++
  PV Panel 5 : Subsystem
  PV Panel 6 : Subsystem
  PV Panel 7 : Subsystem
  PV Panel 8 : Subsystem
  Vout : Outport
  Pout : Outport  Port=2
  wires:
  PV Panel 5/1(Vout) -> Add1/1
  PV Panel 6/2(Pout) -> Add3/2
  PV Panel 7/1(Vout) -> Add1/3
  Wind Speed/1 -> PV Panel 5/3(Wind Speed), PV Panel 6/3(Wind Speed), PV Panel 8/3(Wind Speed), PV Panel 7/3(Wind Speed)
  Tambient/1 -> PV Panel 5/2(Tambient), PV Panel 6/2(Tambient), PV Panel 8/2(Tambient), PV Panel 7/2(Tambient)
  Add3/1 -> Pout/1
  PV Panel 7/2(Pout) -> Add3/3
  lambda_IR/1 -> PV Panel 6/1(Lambda_IR), PV Panel 8/1(Lambda_IR), PV Panel 7/1(Lambda_IR), PV Panel 5/1(Lambda_IR)
  PV Panel 6/1(Vout) -> Add1/2
  PV Panel 8/1(Vout) -> Add1/4
  Add1/1 -> Vout/1
  PV Panel 8/2(Pout) -> Add3/4
  PV Panel 5/2(Pout) -> Add3/1

== system PVRobusMPC_final/4 x 4 x 4 PV Panel 4/4 x 4 PV Panel 6/4 PV Panel 1 ==
  lambda_IR : Inport
  Tambient1 : Inport  Port=2
  Wind Speed : Inport  Port=3
  Add : Sum  Inputs=++++
  Add2 : Sum  Inputs=++++
  PV Panel 1 : Subsystem
  PV Panel 2 : Subsystem
  PV Panel 3 : Subsystem
  PV Panel 4 : Subsystem
  Vout : Outport
  Pout : Outport  Port=2
  wires:
  PV Panel 3/2(Pout) -> Add2/3
  lambda_IR/1 -> PV Panel 1/1(Lambda_IR), PV Panel 2/1(Lambda_IR), PV Panel 4/1(Lambda_IR), PV Panel 3/1(Lambda_IR)
  Add/1 -> Vout/1
  PV Panel 1/2(Pout) -> Add2/1
  Tambient1/1 -> PV Panel 1/2(Tambient), PV Panel 2/2(Tambient), PV Panel 3/2(Tambient), PV Panel 4/2(Tambient)
  PV Panel 1/1(Vout) -> Add/1
  PV Panel 4/1(Vout) -> Add/4
  Wind Speed/1 -> PV Panel 1/3(Wind Speed), PV Panel 2/3(Wind Speed), PV Panel 4/3(Wind Speed), PV Panel 3/3(Wind Speed)
  PV Panel 3/1(Vout) -> Add/3
  PV Panel 2/2(Pout) -> Add2/2
  PV Panel 4/2(Pout) -> Add2/4
  PV Panel 2/1(Vout) -> Add/2
  Add2/1 -> Pout/1

== system PVRobusMPC_final/4 x 4 x 4 PV Panel 4/4 x 4 PV Panel 6/4 PV Panel 2 ==
  lambda_IR : Inport
  Tambient : Inport  Port=2
  Wind Speed : Inport  Port=3
  Add1 : Sum  Inputs=++++
  Add3 : Sum  Inputs=++++
  PV Panel 5 : Subsystem
  PV Panel 6 : Subsystem
  PV Panel 7 : Subsystem
  PV Panel 8 : Subsystem
  Vout : Outport
  Pout : Outport  Port=2
  wires:
  PV Panel 5/1(Vout) -> Add1/1
  PV Panel 6/2(Pout) -> Add3/2
  PV Panel 7/1(Vout) -> Add1/3
  Wind Speed/1 -> PV Panel 5/3(Wind Speed), PV Panel 6/3(Wind Speed), PV Panel 8/3(Wind Speed), PV Panel 7/3(Wind Speed)
  Tambient/1 -> PV Panel 5/2(Tambient), PV Panel 6/2(Tambient), PV Panel 8/2(Tambient), PV Panel 7/2(Tambient)
  Add3/1 -> Pout/1
  PV Panel 7/2(Pout) -> Add3/3
  lambda_IR/1 -> PV Panel 6/1(Lambda_IR), PV Panel 8/1(Lambda_IR), PV Panel 7/1(Lambda_IR), PV Panel 5/1(Lambda_IR)
  PV Panel 6/1(Vout) -> Add1/2
  PV Panel 8/1(Vout) -> Add1/4
  Add1/1 -> Vout/1
  PV Panel 8/2(Pout) -> Add3/4
  PV Panel 5/2(Pout) -> Add3/1

== system PVRobusMPC_final/4 x 4 x 4 PV Panel 4/4 x 4 PV Panel 6/4 PV Panel 3 ==
  lambda_IR : Inport
  Tambient : Inport  Port=2
  Wind Speed : Inport  Port=3
  Add1 : Sum  Inputs=++++
  Add3 : Sum  Inputs=++++
  PV Panel 5 : Subsystem
  PV Panel 6 : Subsystem
  PV Panel 7 : Subsystem
  PV Panel 8 : Subsystem
  Vout : Outport
  Pout : Outport  Port=2
  wires:
  PV Panel 5/2(Pout) -> Add3/1
  PV Panel 8/2(Pout) -> Add3/4
  Add1/1 -> Vout/1
  PV Panel 8/1(Vout) -> Add1/4
  PV Panel 6/1(Vout) -> Add1/2
  lambda_IR/1 -> PV Panel 5/1(Lambda_IR), PV Panel 7/1(Lambda_IR), PV Panel 8/1(Lambda_IR), PV Panel 6/1(Lambda_IR)
  PV Panel 7/2(Pout) -> Add3/3
  Add3/1 -> Pout/1
  Tambient/1 -> PV Panel 7/2(Tambient), PV Panel 8/2(Tambient), PV Panel 6/2(Tambient), PV Panel 5/2(Tambient)
  Wind Speed/1 -> PV Panel 7/3(Wind Speed), PV Panel 8/3(Wind Speed), PV Panel 6/3(Wind Speed), PV Panel 5/3(Wind Speed)
  PV Panel 7/1(Vout) -> Add1/3
  PV Panel 6/2(Pout) -> Add3/2
  PV Panel 5/1(Vout) -> Add1/1

== system PVRobusMPC_final/4 x 4 x 4 PV Panel 4/4 x 4 PV Panel 6/4 PV Panel 4 ==
  lambda_IR : Inport
  Tambient : Inport  Port=2
  Wind Speed : Inport  Port=3
  Add1 : Sum  Inputs=++++
  Add3 : Sum  Inputs=++++
  PV Panel 5 : Subsystem
  PV Panel 6 : Subsystem
  PV Panel 7 : Subsystem
  PV Panel 8 : Subsystem
  Vout : Outport
  Pout : Outport  Port=2
  wires:
  PV Panel 5/1(Vout) -> Add1/1
  PV Panel 6/2(Pout) -> Add3/2
  PV Panel 7/1(Vout) -> Add1/3
  Wind Speed/1 -> PV Panel 5/3(Wind Speed), PV Panel 6/3(Wind Speed), PV Panel 8/3(Wind Speed), PV Panel 7/3(Wind Speed)
  Tambient/1 -> PV Panel 5/2(Tambient), PV Panel 6/2(Tambient), PV Panel 8/2(Tambient), PV Panel 7/2(Tambient)
  Add3/1 -> Pout/1
  PV Panel 7/2(Pout) -> Add3/3
  lambda_IR/1 -> PV Panel 6/1(Lambda_IR), PV Panel 8/1(Lambda_IR), PV Panel 7/1(Lambda_IR), PV Panel 5/1(Lambda_IR)
  PV Panel 6/1(Vout) -> Add1/2
  PV Panel 8/1(Vout) -> Add1/4
  Add1/1 -> Vout/1
  PV Panel 8/2(Pout) -> Add3/4
  PV Panel 5/2(Pout) -> Add3/1

== system PVRobusMPC_final/4 x 4 x 4 PV Panel 4/4 x 4 PV Panel 7/4 PV Panel 1 ==
  lambda_IR : Inport
  Tambient1 : Inport  Port=2
  Wind Speed : Inport  Port=3
  Add : Sum  Inputs=++++
  Add2 : Sum  Inputs=++++
  PV Panel 1 : Subsystem
  PV Panel 2 : Subsystem
  PV Panel 3 : Subsystem
  PV Panel 4 : Subsystem
  Vout : Outport
  Pout : Outport  Port=2
  wires:
  PV Panel 3/2(Pout) -> Add2/3
  lambda_IR/1 -> PV Panel 1/1(Lambda_IR), PV Panel 2/1(Lambda_IR), PV Panel 4/1(Lambda_IR), PV Panel 3/1(Lambda_IR)
  Add/1 -> Vout/1
  PV Panel 1/2(Pout) -> Add2/1
  Tambient1/1 -> PV Panel 1/2(Tambient), PV Panel 2/2(Tambient), PV Panel 3/2(Tambient), PV Panel 4/2(Tambient)
  PV Panel 1/1(Vout) -> Add/1
  PV Panel 4/1(Vout) -> Add/4
  Wind Speed/1 -> PV Panel 1/3(Wind Speed), PV Panel 2/3(Wind Speed), PV Panel 4/3(Wind Speed), PV Panel 3/3(Wind Speed)
  PV Panel 3/1(Vout) -> Add/3
  PV Panel 2/2(Pout) -> Add2/2
  PV Panel 4/2(Pout) -> Add2/4
  PV Panel 2/1(Vout) -> Add/2
  Add2/1 -> Pout/1

== system PVRobusMPC_final/4 x 4 x 4 PV Panel 4/4 x 4 PV Panel 7/4 PV Panel 2 ==
  lambda_IR : Inport
  Tambient : Inport  Port=2
  Wind Speed : Inport  Port=3
  Add1 : Sum  Inputs=++++
  Add3 : Sum  Inputs=++++
  PV Panel 5 : Subsystem
  PV Panel 6 : Subsystem
  PV Panel 7 : Subsystem
  PV Panel 8 : Subsystem
  Vout : Outport
  Pout : Outport  Port=2
  wires:
  PV Panel 5/1(Vout) -> Add1/1
  PV Panel 6/2(Pout) -> Add3/2
  PV Panel 7/1(Vout) -> Add1/3
  Wind Speed/1 -> PV Panel 5/3(Wind Speed), PV Panel 6/3(Wind Speed), PV Panel 8/3(Wind Speed), PV Panel 7/3(Wind Speed)
  Tambient/1 -> PV Panel 5/2(Tambient), PV Panel 6/2(Tambient), PV Panel 8/2(Tambient), PV Panel 7/2(Tambient)
  Add3/1 -> Pout/1
  PV Panel 7/2(Pout) -> Add3/3
  lambda_IR/1 -> PV Panel 6/1(Lambda_IR), PV Panel 8/1(Lambda_IR), PV Panel 7/1(Lambda_IR), PV Panel 5/1(Lambda_IR)
  PV Panel 6/1(Vout) -> Add1/2
  PV Panel 8/1(Vout) -> Add1/4
  Add1/1 -> Vout/1
  PV Panel 8/2(Pout) -> Add3/4
  PV Panel 5/2(Pout) -> Add3/1

== system PVRobusMPC_final/4 x 4 x 4 PV Panel 4/4 x 4 PV Panel 7/4 PV Panel 3 ==
  lambda_IR : Inport
  Tambient : Inport  Port=2
  Wind Speed : Inport  Port=3
  Add1 : Sum  Inputs=++++
  Add3 : Sum  Inputs=++++
  PV Panel 5 : Subsystem
  PV Panel 6 : Subsystem
  PV Panel 7 : Subsystem
  PV Panel 8 : Subsystem
  Vout : Outport
  Pout : Outport  Port=2
  wires:
  PV Panel 5/2(Pout) -> Add3/1
  PV Panel 8/2(Pout) -> Add3/4
  Add1/1 -> Vout/1
  PV Panel 8/1(Vout) -> Add1/4
  PV Panel 6/1(Vout) -> Add1/2
  lambda_IR/1 -> PV Panel 5/1(Lambda_IR), PV Panel 7/1(Lambda_IR), PV Panel 8/1(Lambda_IR), PV Panel 6/1(Lambda_IR)
  PV Panel 7/2(Pout) -> Add3/3
  Add3/1 -> Pout/1
  Tambient/1 -> PV Panel 7/2(Tambient), PV Panel 8/2(Tambient), PV Panel 6/2(Tambient), PV Panel 5/2(Tambient)
  Wind Speed/1 -> PV Panel 7/3(Wind Speed), PV Panel 8/3(Wind Speed), PV Panel 6/3(Wind Speed), PV Panel 5/3(Wind Speed)
  PV Panel 7/1(Vout) -> Add1/3
  PV Panel 6/2(Pout) -> Add3/2
  PV Panel 5/1(Vout) -> Add1/1

== system PVRobusMPC_final/4 x 4 x 4 PV Panel 4/4 x 4 PV Panel 7/4 PV Panel 4 ==
  lambda_IR : Inport
  Tambient : Inport  Port=2
  Wind Speed : Inport  Port=3
  Add1 : Sum  Inputs=++++
  Add3 : Sum  Inputs=++++
  PV Panel 5 : Subsystem
  PV Panel 6 : Subsystem
  PV Panel 7 : Subsystem
  PV Panel 8 : Subsystem
  Vout : Outport
  Pout : Outport  Port=2
  wires:
  PV Panel 5/1(Vout) -> Add1/1
  PV Panel 6/2(Pout) -> Add3/2
  PV Panel 7/1(Vout) -> Add1/3
  Wind Speed/1 -> PV Panel 5/3(Wind Speed), PV Panel 6/3(Wind Speed), PV Panel 8/3(Wind Speed), PV Panel 7/3(Wind Speed)
  Tambient/1 -> PV Panel 5/2(Tambient), PV Panel 6/2(Tambient), PV Panel 8/2(Tambient), PV Panel 7/2(Tambient)
  Add3/1 -> Pout/1
  PV Panel 7/2(Pout) -> Add3/3
  lambda_IR/1 -> PV Panel 6/1(Lambda_IR), PV Panel 8/1(Lambda_IR), PV Panel 7/1(Lambda_IR), PV Panel 5/1(Lambda_IR)
  PV Panel 6/1(Vout) -> Add1/2
  PV Panel 8/1(Vout) -> Add1/4
  Add1/1 -> Vout/1
  PV Panel 8/2(Pout) -> Add3/4
  PV Panel 5/2(Pout) -> Add3/1

== system PVRobusMPC_final/4 x 4 x 4 PV Panel 4/4 x 4 PV Panel 8/4 PV Panel 1 ==
  lambda_IR : Inport
  Tambient1 : Inport  Port=2
  Wind Speed : Inport  Port=3
  Add : Sum  Inputs=++++
  Add2 : Sum  Inputs=++++
  PV Panel 1 : Subsystem
  PV Panel 2 : Subsystem
  PV Panel 3 : Subsystem
  PV Panel 4 : Subsystem
  Vout : Outport
  Pout : Outport  Port=2
  wires:
  Add2/1 -> Pout/1
  PV Panel 2/1(Vout) -> Add/2
  PV Panel 4/2(Pout) -> Add2/4
  PV Panel 2/2(Pout) -> Add2/2
  PV Panel 3/1(Vout) -> Add/3
  Wind Speed/1 -> PV Panel 3/3(Wind Speed), PV Panel 4/3(Wind Speed), PV Panel 2/3(Wind Speed), PV Panel 1/3(Wind Speed)
  PV Panel 4/1(Vout) -> Add/4
  PV Panel 1/1(Vout) -> Add/1
  Tambient1/1 -> PV Panel 4/2(Tambient), PV Panel 3/2(Tambient), PV Panel 2/2(Tambient), PV Panel 1/2(Tambient)
  PV Panel 1/2(Pout) -> Add2/1
  Add/1 -> Vout/1
  lambda_IR/1 -> PV Panel 3/1(Lambda_IR), PV Panel 4/1(Lambda_IR), PV Panel 2/1(Lambda_IR), PV Panel 1/1(Lambda_IR)
  PV Panel 3/2(Pout) -> Add2/3

== system PVRobusMPC_final/4 x 4 x 4 PV Panel 4/4 x 4 PV Panel 8/4 PV Panel 2 ==
  lambda_IR : Inport
  Tambient : Inport  Port=2
  Wind Speed : Inport  Port=3
  Add1 : Sum  Inputs=++++
  Add3 : Sum  Inputs=++++
  PV Panel 5 : Subsystem
  PV Panel 6 : Subsystem
  PV Panel 7 : Subsystem
  PV Panel 8 : Subsystem
  Vout : Outport
  Pout : Outport  Port=2
  wires:
  PV Panel 5/2(Pout) -> Add3/1
  PV Panel 8/2(Pout) -> Add3/4
  Add1/1 -> Vout/1
  PV Panel 8/1(Vout) -> Add1/4
  PV Panel 6/1(Vout) -> Add1/2
  lambda_IR/1 -> PV Panel 5/1(Lambda_IR), PV Panel 7/1(Lambda_IR), PV Panel 8/1(Lambda_IR), PV Panel 6/1(Lambda_IR)
  PV Panel 7/2(Pout) -> Add3/3
  Add3/1 -> Pout/1
  Tambient/1 -> PV Panel 7/2(Tambient), PV Panel 8/2(Tambient), PV Panel 6/2(Tambient), PV Panel 5/2(Tambient)
  Wind Speed/1 -> PV Panel 7/3(Wind Speed), PV Panel 8/3(Wind Speed), PV Panel 6/3(Wind Speed), PV Panel 5/3(Wind Speed)
  PV Panel 7/1(Vout) -> Add1/3
  PV Panel 6/2(Pout) -> Add3/2
  PV Panel 5/1(Vout) -> Add1/1

== system PVRobusMPC_final/4 x 4 x 4 PV Panel 4/4 x 4 PV Panel 8/4 PV Panel 3 ==
  lambda_IR : Inport
  Tambient : Inport  Port=2
  Wind Speed : Inport  Port=3
  Add1 : Sum  Inputs=++++
  Add3 : Sum  Inputs=++++
  PV Panel 5 : Subsystem
  PV Panel 6 : Subsystem
  PV Panel 7 : Subsystem
  PV Panel 8 : Subsystem
  Vout : Outport
  Pout : Outport  Port=2
  wires:
  PV Panel 5/1(Vout) -> Add1/1
  PV Panel 6/2(Pout) -> Add3/2
  PV Panel 7/1(Vout) -> Add1/3
  Wind Speed/1 -> PV Panel 5/3(Wind Speed), PV Panel 6/3(Wind Speed), PV Panel 8/3(Wind Speed), PV Panel 7/3(Wind Speed)
  Tambient/1 -> PV Panel 5/2(Tambient), PV Panel 6/2(Tambient), PV Panel 8/2(Tambient), PV Panel 7/2(Tambient)
  Add3/1 -> Pout/1
  PV Panel 7/2(Pout) -> Add3/3
  lambda_IR/1 -> PV Panel 6/1(Lambda_IR), PV Panel 8/1(Lambda_IR), PV Panel 7/1(Lambda_IR), PV Panel 5/1(Lambda_IR)
  PV Panel 6/1(Vout) -> Add1/2
  PV Panel 8/1(Vout) -> Add1/4
  Add1/1 -> Vout/1
  PV Panel 8/2(Pout) -> Add3/4
  PV Panel 5/2(Pout) -> Add3/1

== system PVRobusMPC_final/4 x 4 x 4 PV Panel 4/4 x 4 PV Panel 8/4 PV Panel 4 ==
  lambda_IR : Inport
  Tambient : Inport  Port=2
  Wind Speed : Inport  Port=3
  Add1 : Sum  Inputs=++++
  Add3 : Sum  Inputs=++++
  PV Panel 5 : Subsystem
  PV Panel 6 : Subsystem
  PV Panel 7 : Subsystem
  PV Panel 8 : Subsystem
  Vout : Outport
  Pout : Outport  Port=2
  wires:
  PV Panel 5/2(Pout) -> Add3/1
  PV Panel 8/2(Pout) -> Add3/4
  Add1/1 -> Vout/1
  PV Panel 8/1(Vout) -> Add1/4
  PV Panel 6/1(Vout) -> Add1/2
  lambda_IR/1 -> PV Panel 5/1(Lambda_IR), PV Panel 7/1(Lambda_IR), PV Panel 8/1(Lambda_IR), PV Panel 6/1(Lambda_IR)
  PV Panel 7/2(Pout) -> Add3/3
  Add3/1 -> Pout/1
  Tambient/1 -> PV Panel 7/2(Tambient), PV Panel 8/2(Tambient), PV Panel 6/2(Tambient), PV Panel 5/2(Tambient)
  Wind Speed/1 -> PV Panel 7/3(Wind Speed), PV Panel 8/3(Wind Speed), PV Panel 6/3(Wind Speed), PV Panel 5/3(Wind Speed)
  PV Panel 7/1(Vout) -> Add1/3
  PV Panel 6/2(Pout) -> Add3/2
  PV Panel 5/1(Vout) -> Add1/1

== system PVRobusMPC_final/4 x 4 x 4 PV Panel 1/4 x 4 PV Panel 1/4 PV Panel 1/PV Panel 1 ==
  Lambda_IR : Inport
  Tambient : Inport  Port=2
  Wind Speed : Inport  Port=3
  PV MPC : Subsystem
  Photovolatic Panel : Subsystem  mask{Temp_Initial=380}
      mask prompts: Temp_Initial "Initial Temperature in C"
  To Workspace : ToWorkspace  VariableName=Tm_f01  SampleTime=1
  To Workspace1 : ToWorkspace  VariableName=Pout01  SampleTime=1
  To Workspace2 : ToWorkspace  VariableName=Lambda_UV01  SampleTime=1
  Unit Delay : UnitDelay  InitialCondition=380
  Unit Delay1 : UnitDelay  InitialCondition=4
  Vout : Outport
  Pout : Outport  Port=2
  wires:
  Unit Delay/1 -> PV MPC/1(Tm_f), To Workspace/1
  PV MPC/1(Lambda_UV) -> To Workspace2/1, Photovolatic Panel/1(Lambda_UV)
  Unit Delay1/1 -> Pout/1, To Workspace1/1
  Lambda_IR/1 -> Photovolatic Panel/2(Lambda_IR)
  Photovolatic Panel/3(Vout [Volts]) -> Vout/1
  Tambient/1 -> PV MPC/2(Tambient), Photovolatic Panel/3(Tambient)
  Photovolatic Panel/2(Pout [Watt]) -> Unit Delay1/1
  Photovolatic Panel/1(Tm_f [K]) -> Unit Delay/1
  Wind Speed/1 -> Photovolatic Panel/4(WS)

== system PVRobusMPC_final/4 x 4 x 4 PV Panel 1/4 x 4 PV Panel 1/4 PV Panel 1/PV Panel 2 ==
  Lambda_IR : Inport
  Tambient : Inport  Port=2
  Wind Speed : Inport  Port=3
  PV MPC : Subsystem
  Photovolatic Panel : Subsystem  mask{Temp_Initial=380}
      mask prompts: Temp_Initial "Initial Temperature in C"
  Unit Delay : UnitDelay  InitialCondition=380
  Unit Delay1 : UnitDelay  InitialCondition=4
  Vout : Outport
  Pout : Outport  Port=2
  wires:
  Wind Speed/1 -> Photovolatic Panel/4(WS)
  Photovolatic Panel/1(Tm_f [K]) -> Unit Delay/1
  Photovolatic Panel/2(Pout [Watt]) -> Unit Delay1/1
  Tambient/1 -> Photovolatic Panel/3(Tambient), PV MPC/2(Tambient)
  Photovolatic Panel/3(Vout [Volts]) -> Vout/1
  Lambda_IR/1 -> Photovolatic Panel/2(Lambda_IR)
  Unit Delay1/1 -> Pout/1
  PV MPC/1(Lambda_UV) -> Photovolatic Panel/1(Lambda_UV)
  Unit Delay/1 -> PV MPC/1(Tm_f)

== system PVRobusMPC_final/4 x 4 x 4 PV Panel 1/4 x 4 PV Panel 1/4 PV Panel 1/PV Panel 3 ==
  Lambda_IR : Inport
  Tambient : Inport  Port=2
  Wind Speed : Inport  Port=3
  PV MPC : Subsystem
  Photovolatic Panel : Subsystem  mask{Temp_Initial=380}
      mask prompts: Temp_Initial "Initial Temperature in C"
  Unit Delay : UnitDelay  InitialCondition=380
  Unit Delay1 : UnitDelay  InitialCondition=4
  Vout : Outport
  Pout : Outport  Port=2
  wires:
  Unit Delay/1 -> PV MPC/1(Tm_f)
  PV MPC/1(Lambda_UV) -> Photovolatic Panel/1(Lambda_UV)
  Unit Delay1/1 -> Pout/1
  Lambda_IR/1 -> Photovolatic Panel/2(Lambda_IR)
  Photovolatic Panel/3(Vout [Volts]) -> Vout/1
  Tambient/1 -> PV MPC/2(Tambient), Photovolatic Panel/3(Tambient)
  Photovolatic Panel/2(Pout [Watt]) -> Unit Delay1/1
  Photovolatic Panel/1(Tm_f [K]) -> Unit Delay/1
  Wind Speed/1 -> Photovolatic Panel/4(WS)

== system PVRobusMPC_final/4 x 4 x 4 PV Panel 1/4 x 4 PV Panel 1/4 PV Panel 1/PV Panel 4 ==
  Lambda_IR : Inport
  Tambient : Inport  Port=2
  Wind Speed : Inport  Port=3
  PV MPC : Subsystem
  Photovolatic Panel : Subsystem  mask{Temp_Initial=380}
      mask prompts: Temp_Initial "Initial Temperature in C"
  Unit Delay : UnitDelay  InitialCondition=380
  Unit Delay1 : UnitDelay  InitialCondition=4
  Vout : Outport
  Pout : Outport  Port=2
  wires:
  Wind Speed/1 -> Photovolatic Panel/4(WS)
  Photovolatic Panel/1(Tm_f [K]) -> Unit Delay/1
  Photovolatic Panel/2(Pout [Watt]) -> Unit Delay1/1
  Tambient/1 -> Photovolatic Panel/3(Tambient), PV MPC/2(Tambient)
  Photovolatic Panel/3(Vout [Volts]) -> Vout/1
  Lambda_IR/1 -> Photovolatic Panel/2(Lambda_IR)
  Unit Delay1/1 -> Pout/1
  PV MPC/1(Lambda_UV) -> Photovolatic Panel/1(Lambda_UV)
  Unit Delay/1 -> PV MPC/1(Tm_f)

== system PVRobusMPC_final/4 x 4 x 4 PV Panel 1/4 x 4 PV Panel 1/4 PV Panel 2/PV Panel 5 ==
  Lambda_IR : Inport
  Tambient : Inport  Port=2
  Wind Speed : Inport  Port=3
  PV MPC : Subsystem
  Photovolatic Panel : Subsystem  mask{Temp_Initial=380}
      mask prompts: Temp_Initial "Initial Temperature in C"
  Unit Delay : UnitDelay  InitialCondition=380
  Unit Delay1 : UnitDelay  InitialCondition=4
  Vout : Outport
  Pout : Outport  Port=2
  wires:
  Unit Delay/1 -> PV MPC/1(Tm_f)
  PV MPC/1(Lambda_UV) -> Photovolatic Panel/1(Lambda_UV)
  Unit Delay1/1 -> Pout/1
  Lambda_IR/1 -> Photovolatic Panel/2(Lambda_IR)
  Photovolatic Panel/3(Vout [Volts]) -> Vout/1
  Tambient/1 -> PV MPC/2(Tambient), Photovolatic Panel/3(Tambient)
  Photovolatic Panel/2(Pout [Watt]) -> Unit Delay1/1
  Photovolatic Panel/1(Tm_f [K]) -> Unit Delay/1
  Wind Speed/1 -> Photovolatic Panel/4(WS)

== system PVRobusMPC_final/4 x 4 x 4 PV Panel 1/4 x 4 PV Panel 1/4 PV Panel 2/PV Panel 6 ==
  Lambda_IR : Inport
  Tambient : Inport  Port=2
  Wind Speed : Inport  Port=3
  PV MPC : Subsystem
  Photovolatic Panel : Subsystem  mask{Temp_Initial=380}
      mask prompts: Temp_Initial "Initial Temperature in C"
  Unit Delay : UnitDelay  InitialCondition=380
  Unit Delay1 : UnitDelay  InitialCondition=4
  Vout : Outport
  Pout : Outport  Port=2
  wires:
  Wind Speed/1 -> Photovolatic Panel/4(WS)
  Photovolatic Panel/1(Tm_f [K]) -> Unit Delay/1
  Photovolatic Panel/2(Pout [Watt]) -> Unit Delay1/1
  Tambient/1 -> Photovolatic Panel/3(Tambient), PV MPC/2(Tambient)
  Photovolatic Panel/3(Vout [Volts]) -> Vout/1
  Lambda_IR/1 -> Photovolatic Panel/2(Lambda_IR)
  Unit Delay1/1 -> Pout/1
  PV MPC/1(Lambda_UV) -> Photovolatic Panel/1(Lambda_UV)
  Unit Delay/1 -> PV MPC/1(Tm_f)

== system PVRobusMPC_final/4 x 4 x 4 PV Panel 1/4 x 4 PV Panel 1/4 PV Panel 2/PV Panel 7 ==
  Lambda_IR : Inport
  Tambient : Inport  Port=2
  Wind Speed : Inport  Port=3
  PV MPC : Subsystem
  Photovolatic Panel : Subsystem  mask{Temp_Initial=380}
      mask prompts: Temp_Initial "Initial Temperature in C"
  Unit Delay : UnitDelay  InitialCondition=380
  Unit Delay1 : UnitDelay  InitialCondition=4
  Vout : Outport
  Pout : Outport  Port=2
  wires:
  Unit Delay/1 -> PV MPC/1(Tm_f)
  PV MPC/1(Lambda_UV) -> Photovolatic Panel/1(Lambda_UV)
  Unit Delay1/1 -> Pout/1
  Lambda_IR/1 -> Photovolatic Panel/2(Lambda_IR)
  Photovolatic Panel/3(Vout [Volts]) -> Vout/1
  Tambient/1 -> PV MPC/2(Tambient), Photovolatic Panel/3(Tambient)
  Photovolatic Panel/2(Pout [Watt]) -> Unit Delay1/1
  Photovolatic Panel/1(Tm_f [K]) -> Unit Delay/1
  Wind Speed/1 -> Photovolatic Panel/4(WS)
